simulink model "QpskRxBradeRf"  (R2015b)
settings: Solver=VariableStepAuto  StartTime=0.0  StopTime=inf  RelTol=1e-3
InitFcn:
  | % General simulation parameters
  | M = 4;                         % M-PSK alphabet size
  | Upsampling = 4;            % Upsampling factor
  | Downsampling = 2;        % Downsampling factor
  | Fs = 2e6;                     % Sample rate
  | Ts = 1/Fs;                    % Sample time
  | FrameSize = 111;          % Number of modulated symbols per frame
  | %MessageLength = 105;  % Number of message bits per frame, 7 ASCII characters
  | BarkerLength = 13;        % Number of Barker code symbols
  | 
  | % Rx parameters
  | K = 1;
  | A = 1/sqrt(2);
  | 
  | % TED
  | %fs = 2.4e6;
  | %fs = Fs/2;
  | fs = Fs;
  | Rdata = 100e3;
  | Rsymbol = Rdata/2;
  | 
  | % --- Early Late Timing Synchronisation ----
  | % synch loop design
  | d = 0.707;                   % damping ratio
  | 
  | %Ts = 1/Rsymbol;           % symbol period
  | Ks = 3.22;                    % phase detector coefficient
  | BnS = 0.1*Rsymbol;      % noise bandwidth in Hz
  | Kn   = 1;                      % gain of numerically controlled clock
  | 
  | % calculate loop filter coefficients
  | Ka = (4*d*BnS*Ts)/(Kn*Ks*(d+1/(4*d)));
  | Kb = (4*(BnS*Ts)^2)/(Kn*Ks*(d+1/4*d)^2);
  | 
  | % ------- Carrier Synchronisation --------
  | T = 1/fs;       % sample period
  | Kp = 1;          % phase detector S-curve is linear
  | Bn = 25000;   % noise bandwidth in Hz
  | Ko = 1;          % gain of NCO (here just a direct conversion)
  | 
  | d = 0.707;  % damping ratio
  | 
  | % calculate the loop filter coefficients
  | K1 = (4*d*Bn*T)/(Ko*Kp*(d+1/(4*d)));
  | K2 = (4*(Bn*T)^2)/(Ko*Kp*(d+1/4*d)^2);
libraries: simulink x5, dspstat3 x3, commdigbbndpm3 x2, commrfcorlib x1, commrflib2 x1, commblksprivate x1, dspspect3 x1, commsequence2 x1, dspsigops x1, commutil2 x1, commfilt2 x1
settings Model: ModifiedByFormat=RapidRadio  Creator=RapidRadio  LastModifiedBy=RapidRadio

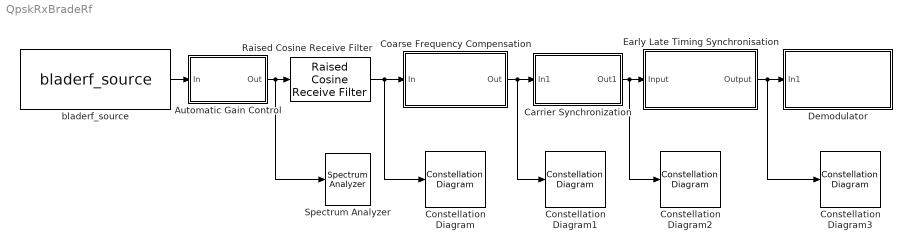
== system QpskRxBradeRf ==
  Automatic Gain Control : Subsystem  mask{DesiredAmplitude=1/sqrt(Upsampling)}
      mask prompts: DesiredAmplitude "Desired Amplitude"
      mask Display: disp('Automatic Gain\nControl')
  Carrier Synchronization : Subsystem
      mask Display: disp('Carrier\nSynchronization');
  Coarse Frequency Compensation : Subsystem
      mask Display: disp('Coarse Frequency\nCompensation');
  Constellation Diagram{,1..3} (4 alike) : ConstellationDiagram
  Demodulator : Subsystem
      mask Display: disp('Demodulator');
  Early Late Timing Synchronisation : Subsystem
      mask Display: disp('Early Late Timing\nSynchronisation');
  Raised Cosine Receive Filter : commfilt2/Raised Cosine Receive Filter  filtType=Square root  N=8  filtSpan=10  currentFiltSpan=10  D=(10)/2  R=0.5  sampMode=Mute  saveAsFlag=0  rateMode=Downsampling  downFactor=8  downOffset=1  framing=Enforce single-rate processing  InputProcessing=Columns as channels (frame based)  checkGain=Normalized  filterGain=1  checkCoeff=off  variableName=rcRxFilt1  launchFVT=off  roundingMode=Floor  overflowMode=off
  Spectrum Analyzer : SpectrumAnalyzer
  bladerf_source : S-Function  FunctionName=bladerf_source  Parameters=set_index,samplerate,set_bandwidth,set_freq,set_lnagain,set_rxvga1,set_rxvga2,set_frame,set_frame_type  SFunctionDeploymentMode=off  EnableBusSupport=off  mask(bladeRF Source){bladerf_device_index=0, bladerf_query=off, bladerf_samplerate=2e6, bladerf_lpf=1.75 MHz, bladerf_frame_length=888, bladerf_frame_type=Frame, bladerf_frequency=2.4e9, bladerf_rxlna=6dB, bladerf_rxvga1=10, bladerf_rxvga2=10, bladerf_restore_block=off}
      mask prompts: bladerf_device_index "Device Index:"; bladerf_query "Find Devices (click, see MATLAB console output)"; bladerf_samplerate "Sample Rate (SPS):"; bladerf_lpf "Low Pass Filter Bandwidth:"; bladerf_frame_length "Samples per frame"; bladerf_frame_type "Output Type:"; bladerf_frequency "Carrier Frequency (Hz):"; bladerf_rxlna "RXLNA Gain (dB)"; bladerf_rxvga1 "RXVGA1 Gain (dB)"; bladerf_rxvga2 "RXVGA2 Gain (dB)"; bladerf_restore_block "Restore Block Size (click)"
      mask help: Receive data from a bladeRF device.
      mask init:
      | % initialize
      | % S-params set_index,samplerate,set_bandwidth,set_freq,set_lnagain,set_rxvga1,set_rxvga2,set_frame,set_frame_type
      | mask_display_text = [];
      | 
      | port=0;
      | % check identifier
      | if (isreal(bladerf_device_index) && bladerf_device_index >= 0)
      |     set_index=bladerf_device_index;
      | else
      |     error('The device index must be a number greater or equal 0 !!!')
      | end
      | 
      | % mask display device index
      | if strcmp(get_param(gcb,'bladerf_device_index'),' ')
      |     mask_display_text = [mask_display_text 'disp(''No Device'');'];
      | else
      |     mask_display_text = [mask_display_text 'disp(''bladeRF #' num2str(bladerf_device_index) ''');'];
      | end
      | if (bladerf_samplerate < bladerf_lpf)
      |     warning('The bandwidth should be lower than the samplerate, use with caution')
      | end
      | % check samplerate
      | if (isreal(bladerf_samplerate))
      |     if (bladerf_samplerate > 0)
      |         samplerate=uint32(bladerf_samplerate);
      |         if (samplerate ~= bladerf_samplerate)
      |             fprintf('Sample Rate adjusted to %u Sps\n',samplerate);
      |         end
      |     else
      |         error('The samplerate has to be greater than 0 !!!')
      |     end
      | else
      |     error('The samplerate has to be number !!!')
      | end
      | 
      | bws = [28e6 20e6 14e6 12e6 8.75e6 7e6 6e6 5.5e6 5e6 3.84e6 3e6 2.75e6 2.5e6 1.75e6 1.5e6];
      | set_bandwidth = bws(bladerf_lpf);
      | if (set_bandwidth > bladerf_samplerate)
      |     warning('Sampling rate (Sps) should be equal to or greater than Low Pass Filter Bandwidth to satisfy Nyquist sampling rate');
      | end
      | 
      | % check frequency
      | if (isreal(bladerf_frequency) && bladerf_frequency >= 0)
      |         set_freq=uint32(bladerf_frequency);
      |         if (set_freq ~= bladerf_frequency)
      |                 fprintf('Frequency adjusted to %d\n',set_freq);
      |         end
      | else
      |     error('The frequency has to be number greater than 0 !!!')
      | end
      | 
      | % LNA gain
      | if (isreal(bladerf_rxlna))
      |     if (bladerf_rxlna == 0)
      |         set_lnagain = 6;
      |     elseif (bladerf_rxlna == 1)
      |         set_lnagain = 3;
      |     else
      |         set_lnagain = 0;
      |     end
      | end
      | 
      | % RXVGA1
      | if (isreal(bladerf_rxvga1))
      |     if (bladerf_rxvga1 < 5)
      |         error('RXVGA1 Gain has to be greater than or equal to 5dB\n');
      |     elseif (bladerf_rxvga1 > 30)
      |         error('RXVGA1 Gain has to be less than or equal to 30dB\n');
      |     else
      |         set_rxvga1 = uint32(bladerf_rxvga1);
      |         if (set_rxvga1 ~= bladerf_rxvga1)
      |             fprintf('RXVGA1 Gain set to %u dB\n', set_rxvga1)
      |         end
      |     end
      | end
      | 
      | % RXVGA2
      | if (isreal(bladerf_rxvga2))
      |     if (bladerf_rxvga2 < 0)
      |         error('RXVGA2 Gain has to be greater than or equal to 0dB\n');
      |     elseif (bladerf_rxvga2 > 30)
      |         error('RXVGA2 Gain has to be less than or equal to 30dB\n');
      |     else
      |         set_rxvga2 = uint32(bladerf_rxvga2);
      |         if (set_rxvga2 ~= bladerf_rxvga2)
      |             fprintf('RXVGA2 Gain set to %u dB\n', set_rxvga2)
      |         end
      |     end
      | end
      | 
      | % check frame length
      | if (isreal(bladerf_frame_length) && bladerf_frame_length > 0)
      |     set_frame=bladerf_frame_length;
      | else
      |     error('The frame length has to be number greater than 0 !!!')
      | end
      | 
      | % check frame type
      | if (strcmp(get_param(gcb,'bladerf_frame_type'),'Frame'))
      |     % use frames
      |     set_frame_type=1;
      | else
      |     % use vectors
      |     set_frame_type=0;
      | end
      |     
      | % set mask display
      | set_param(gcb,'MaskDisplay',mask_display_text);
      mask Help: web(fullfile(bladerf_get_path, 'blockset', 'bladerf_source.html'), '-helpbrowser')
      mask Callback bladerf_query:
      | stat=get_param(gcb,'bladerf_query');
      | set_param(gcb,'bladerf_query','off');
      | 
      | if strcmp(stat,'on')
      |     clear stat;
      |     bladerf_find_devices;
      | end
      | 
      | clear stat;
      mask TypeOptions bladerf_lpf: 28 MHz | 20 MHz | 14 Mhz | 12 Mhz | 8.75 Mhz | 7 MHz | 6 Mhz | 5.5 MHz | 5 MHz | 3.84 MHz | 3 MHz | 2.75 MHz | 2.5 MHz | 1.75 MHz | 1.5 MHz
      mask TypeOptions bladerf_frame_type: Frame | Vector
      mask TypeOptions bladerf_rxlna: 6dB | 3dB | 0dB
      mask Callback bladerf_restore_block:
      | % restore block size
      | block_width=150;
      | block_height=60;
      | 
      | if strcmp(get_param(gcb,'bladerf_restore_block'),'on')
      |    pos=get_param(gcb,'Position');
      |    pos=[pos(1) pos(2) pos(1)+block_width pos(2)+block_height];
      |    set_param(gcb,'Position',pos);
      | end
      | 
      | set_param(gcb,'bladerf_restore_block','off');
      | 
      | clear pos block_width block_height
      mask Display: disp('bladeRF #0');
  wires:
  Raised Cosine Receive Filter/1 -> Constellation Diagram/1, Coarse Frequency Compensation/1(In)
  bladerf_source/1 -> Automatic Gain Control/1(In)
  Coarse Frequency Compensation/1(Out) -> Carrier Synchronization/1(In1), Constellation Diagram1/1
  Early Late Timing Synchronisation/1(Output) -> Demodulator/1(In1), Constellation Diagram3/1
  Automatic Gain Control/1(Out) -> Raised Cosine Receive Filter/1, Spectrum Analyzer/1
  Carrier Synchronization/1(Out1) -> Early Late Timing Synchronisation/1(Input), Constellation Diagram2/1

== system QpskRxBradeRf/Automatic Gain Control ==
  In : Inport
  AGC : commrfcorlib/AGC  LegacyMode=off  DetectorMethod=Rectifier  LoopMethod=Linear  UpdatePeriod=40  StepSize=0.1  AdaptationStepSize=(0.1)/(40)  DesiredOutputPower=1  AveragingLength=40  MaximumGain=1e6  MaxPowerGain=2*(1e6)  GainOutputPort=off  InputPowerOutputPort=off  SimulateUsing=Code generation
  Gain : Gain  Gain=DesiredAmplitude
  Out : Outport
  wires:
  In/1 -> AGC/1
  AGC/1 -> Gain/1
  Gain/1 -> Out/1

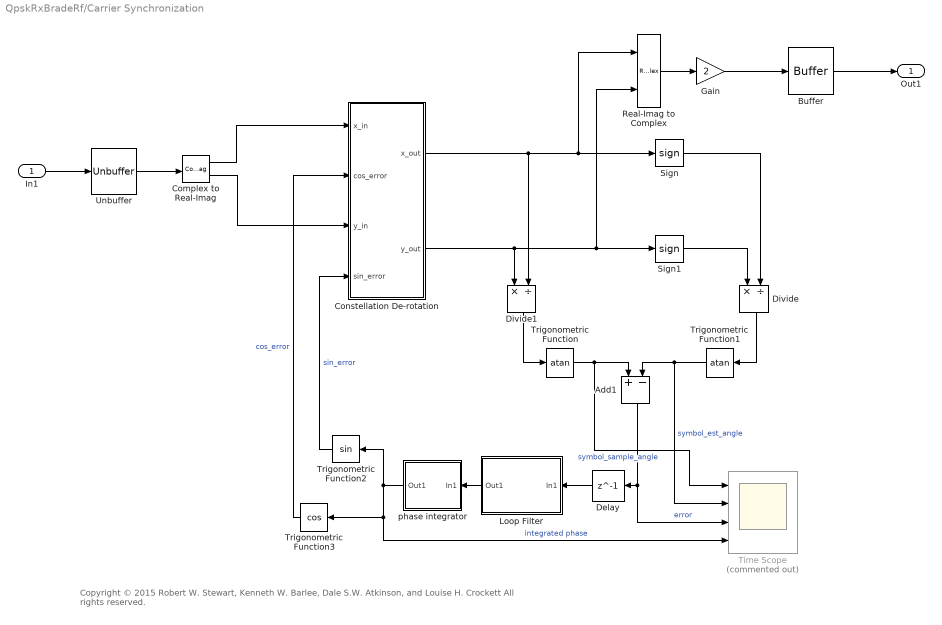
== system QpskRxBradeRf/Carrier Synchronization ==
  note: Copyright © 2015 Robert W. Stewart, Kenneth W. Barlee, Dale S.W. Atkinson, and Louise H. Crockett All rights reserved.
  In1 : Inport
  Add1 : Sum  Inputs=+-
  Buffer : Buffer  N=111  TreatMby1Signals=One channel  OutputFrames=off
  Complex to Real-Imag : ComplexToRealImag
  Constellation De-rotation : Subsystem
  Delay : Delay  DelayLength=1
  Divide : Product  Inputs=*/
  Divide1 : Product  Inputs=*/
  Gain : Gain  Gain=2
  Loop Filter : Subsystem
  Real-Imag to Complex : RealImagToComplex
  Sign : Signum
  Sign1 : Signum
  Time Scope : Scope  Commented=on  NumInputPorts=4
      settings: StartFcn=startfcn_time_scope;
  Trigonometric Function : Trigonometry  Operator=atan  OutputSignalType=real
  Trigonometric Function1 : Trigonometry  Operator=atan  OutputSignalType=real
  Trigonometric Function2 : Trigonometry
  Trigonometric Function3 : Trigonometry  Operator=cos
  Unbuffer : Unbuffer  SampleBasedProcessing=Same as frame based
  phase integrator : Subsystem
  Out1 : Outport
  wires:
  Real-Imag to Complex/1 -> Gain/1
  Sign1/1 -> Divide/1
  Sign/1 -> Divide/2
  Constellation De-rotation/2(y_out) -> Sign1/1, Real-Imag to Complex/2, Divide1/1
  Divide/1 -> Trigonometric Function1/1
  Delay/1 -> Loop Filter/1(In1)
  Divide1/1 -> Trigonometric Function/1
  Add1/1 -> Time Scope/3, Delay/1  "error"
  Constellation De-rotation/1(x_out) -> Sign/1, Real-Imag to Complex/1, Divide1/2
  phase integrator/1(Out1) -> Trigonometric Function2/1, Time Scope/4, Trigonometric Function3/1  "integrated phase"
  Trigonometric Function1/1 -> Time Scope/2, Add1/2  "symbol_est_angle"
  Trigonometric Function/1 -> Add1/1, Time Scope/1  "symbol_sample_angle"
  Trigonometric Function2/1 -> Constellation De-rotation/4(sin_error)  "sin_error"
  Trigonometric Function3/1 -> Constellation De-rotation/2(cos_error)  "cos_error"
  Loop Filter/1(Out1) -> phase integrator/1(In1)
  Complex to Real-Imag/1 -> Constellation De-rotation/1(x_in)
  Complex to Real-Imag/2 -> Constellation De-rotation/3(y_in)
  In1/1 -> Unbuffer/1
  Unbuffer/1 -> Complex to Real-Imag/1
  Gain/1 -> Buffer/1
  Buffer/1 -> Out1/1

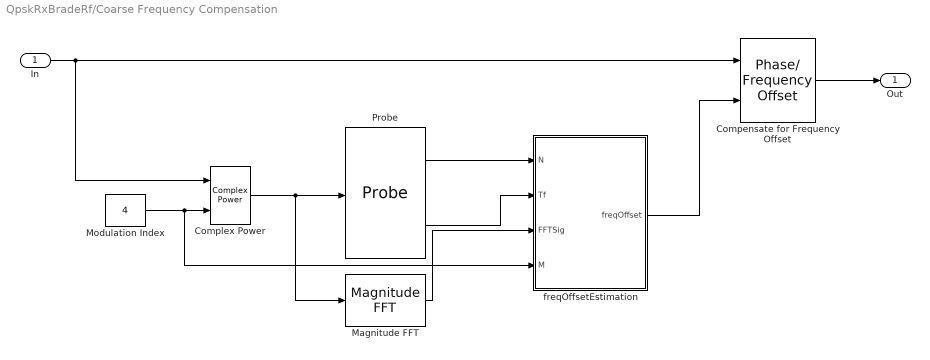
== system QpskRxBradeRf/Coarse Frequency Compensation ==
  In : Inport
  Compensate for Frequency Offset : commrflib2/Phase// Frequency Offset  phaseOffset=0  freqPort=on  freqOffset=100
  Complex Power : commblksprivate/Complex Power
  Magnitude FFT : dspspect3/Magnitude FFT  mag_or_magsq=Magnitude squared  FFTImplementation=Auto  fftLenInherit=on  fftsize=1024  WrapInput=on
  Modulation Index : Constant  Value=4  OutDataTypeStr=Inherit: Inherit via back propagation
  Probe : Probe  ProbeComplexSignal=off
  freqOffsetEstimation : MATLAB Function  TreatAsAtomicUnit=on
  Out : Outport
  wires:
  Compensate for Frequency Offset/1 -> Out/1
  freqOffsetEstimation/1(freqOffset) -> Compensate for Frequency Offset/2
  Magnitude FFT/1 -> freqOffsetEstimation/3(FFTSig)
  Modulation Index/1 -> freqOffsetEstimation/4(M), Complex Power/2
  Probe/1 -> freqOffsetEstimation/1(N)
  Probe/2 -> freqOffsetEstimation/2(Tf)
  Complex Power/1 -> Magnitude FFT/1, Probe/1
  In/1 -> Complex Power/1, Compensate for Frequency Offset/1

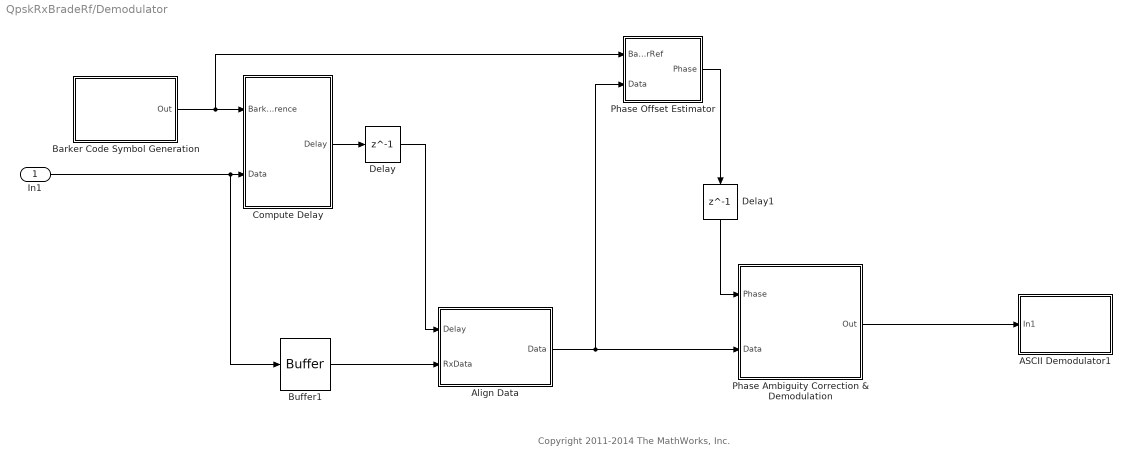
== system QpskRxBradeRf/Demodulator ==
  note: Copyright 2011-2014 The MathWorks, Inc.
  In1 : Inport
  ASCII Demodulator1 : Subsystem
      mask Display: disp('ASCII Demodulator')
  Align Data : MATLAB Function  TreatAsAtomicUnit=on
  "Barker Code Symbol Generation " : Subsystem
      mask Display: disp('Barker Code\nSymbol Generation')
  Buffer1 : Buffer  N=FrameSize*2  V=FrameSize  TreatMby1Signals=One channel
  Compute Delay : Subsystem
      mask Display: disp('Compute\nDelay');
  Delay : Delay  DelayLength=1
  Delay1 : Delay  DelayLength=1
  Phase Ambiguity Correction & Demodulation : Subsystem
      mask Display: disp('Phase Ambiguity\nCorrection\n& Demodulation');
  Phase Offset Estimator : Subsystem
  wires:
  In1/1 -> Buffer1/1, Compute Delay/2(Data)
  Delay/1 -> Align Data/1(Delay)
  Compute Delay/1(Delay) -> Delay/1
  Align Data/1(Data) -> Phase Ambiguity Correction & Demodulation/2(Data), Phase Offset Estimator/2(Data)
  "Barker Code Symbol Generation "/1(Out) -> Compute Delay/1(Barker Reference), Phase Offset Estimator/1(BarkerRef)
  Buffer1/1 -> Align Data/2(RxData)
  Phase Offset Estimator/1(Phase) -> Delay1/1
  Delay1/1 -> Phase Ambiguity Correction & Demodulation/1(Phase)
  Phase Ambiguity Correction & Demodulation/1(Out) -> ASCII Demodulator1/1(In1)

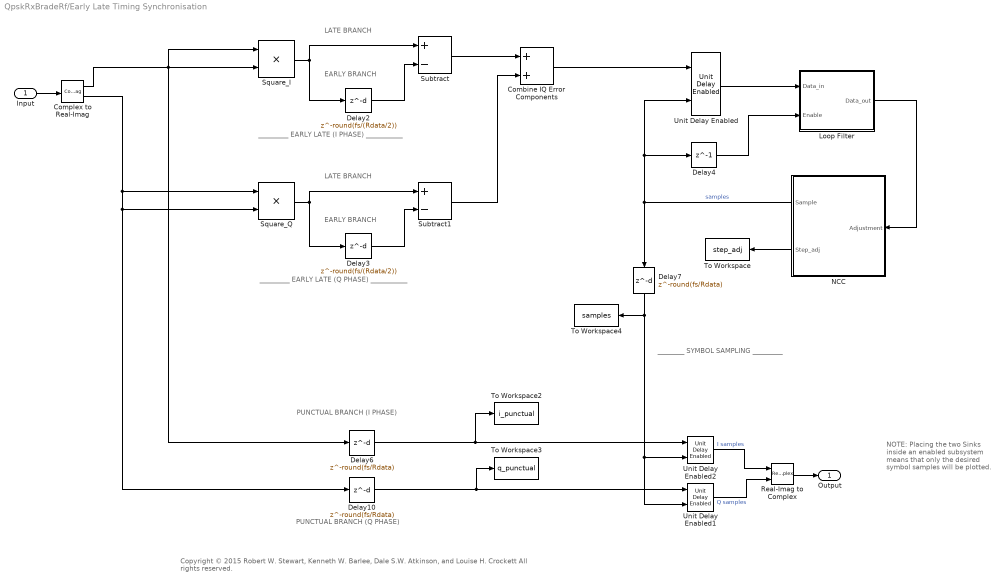
== system QpskRxBradeRf/Early Late Timing Synchronisation ==
  note: NOTE:
      |
      | Placing the two Sinks inside an
      | enabled subsystem means that
      | only the desired symbol samples
      | will be plotted.
  note: LATE BRANCH
  note: EARLY BRANCH
  note: PUNCTUAL BRANCH (I PHASE)
  note: LATE BRANCH
  note: EARLY BRANCH
  note: _________ EARLY LATE (I PHASE) ___________
  note: _________ EARLY LATE (Q PHASE) ___________
  note: ________ SYMBOL SAMPLING _________
  note: PUNCTUAL BRANCH (Q PHASE)
  note: Copyright © 2015 Robert W. Stewart, Kenneth W. Barlee, Dale S.W. Atkinson, and Louise H. Crockett All rights reserved.
  Input : Inport
  Combine IQ Error Components : Sum
  Complex to Real-Imag : ComplexToRealImag
  Delay10 : Delay  DelayLength=round(fs/Rdata)
  Delay2 : Delay  DelayLength=round(fs/(Rdata/2))
  Delay3 : Delay  DelayLength=round(fs/(Rdata/2))
  Delay4 : Delay  DelayLength=1
  Delay6 : Delay  DelayLength=round(fs/Rdata)
  Delay7 : Delay  DelayLength=round(fs/Rdata)
  Loop Filter : Subsystem
  NCC : Subsystem  mask(Numerically Controller Clock (NCC)){OSR=fs/Rsymbol}
      mask prompts: OSR "Oversampling Ratio"
      mask help:
      | This component operates similarly to a Numerically Controlled Oscillator (NCO).
      |
      | Internally, a nominal step size of (1 + Adjustment) is applied to an accumulator. The accumulator wraps around at N = OSR, therefore for a zero control input, the accumulator wraps once every symbol period at the expected rate.
      |
      | When the accumulator wraps, a strobe output is produced.
  Real-Imag to Complex : RealImagToComplex
  Square_I : Product
  Square_Q : Product
  Subtract : Sum  Inputs=+-
  Subtract1 : Sum  Inputs=+-
  To Workspace : ToWorkspace  VariableName=step_adj  SaveFormat=Structure With Time  SampleTime=-1
  To Workspace2 : ToWorkspace  VariableName=i_punctual  SaveFormat=Structure With Time  SampleTime=-1
  To Workspace3 : ToWorkspace  VariableName=q_punctual  SaveFormat=Structure With Time  SampleTime=-1
  To Workspace4 : ToWorkspace  VariableName=samples  SaveFormat=Structure With Time  SampleTime=-1
  Unit Delay Enabled : simulink/Additional Math & Discrete/Additional Discrete/Unit Delay Enabled  vinit=0.0  tsamp=-1
  Unit Delay Enabled1 : simulink/Additional Math & Discrete/Additional Discrete/Unit Delay Enabled  vinit=0.0  tsamp=-1
  Unit Delay Enabled2 : simulink/Additional Math & Discrete/Additional Discrete/Unit Delay Enabled  vinit=0.0  tsamp=-1
  Output : Outport
  wires:
  Subtract/1 -> Combine IQ Error Components/1
  Delay4/1 -> Loop Filter/2(Enable)
  Square_Q/1 -> Delay3/1, Subtract1/1
  Square_I/1 -> Subtract/1, Delay2/1
  Delay2/1 -> Subtract/2
  Unit Delay Enabled/1 -> Loop Filter/1(Data_in)
  NCC/1(Sample) -> Unit Delay Enabled/2, Delay4/1, Delay7/1  "samples"
  Loop Filter/1(Data_out) -> NCC/1(Adjustment)
  Subtract1/1 -> Combine IQ Error Components/2
  Complex to Real-Imag/1 -> Square_I/1, Delay6/1, Square_I/2
  Delay6/1 -> To Workspace2/1, Unit Delay Enabled2/1
  Delay3/1 -> Subtract1/2
  Unit Delay Enabled2/1 -> Real-Imag to Complex/1  "I samples"
  NCC/2(Step_adj) -> To Workspace/1
  Combine IQ Error Components/1 -> Unit Delay Enabled/1
  Unit Delay Enabled1/1 -> Real-Imag to Complex/2  "Q samples"
  Delay10/1 -> To Workspace3/1, Unit Delay Enabled1/1
  Complex to Real-Imag/2 -> Delay10/1, Square_Q/2, Square_Q/1
  Delay7/1 -> Unit Delay Enabled2/2, Unit Delay Enabled1/2, To Workspace4/1
  Input/1 -> Complex to Real-Imag/1
  Real-Imag to Complex/1 -> Output/1

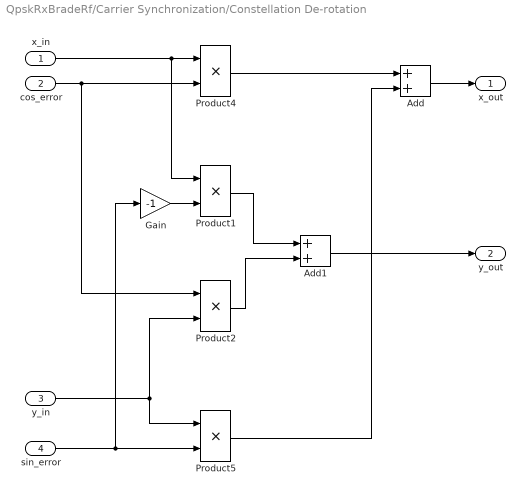
== system QpskRxBradeRf/Carrier Synchronization/Constellation De-rotation ==
  x_in : Inport
  cos_error : Inport  Port=2
  y_in : Inport  Port=3
  sin_error : Inport  Port=4
  Add : Sum
  Add1 : Sum
  Gain : Gain  Gain=-1
  Product{1..2,4..5} (4 alike) : Product
  x_out : Outport
  y_out : Outport  Port=2
  wires:
  Product4/1 -> Add/1
  y_in/1 -> Product2/2, Product5/1
  sin_error/1 -> Gain/1, Product5/2
  x_in/1 -> Product1/1, Product4/1
  Product5/1 -> Add/2
  cos_error/1 -> Product2/1, Product4/2
  Add/1 -> x_out/1
  Gain/1 -> Product1/2
  Product2/1 -> Add1/2
  Product1/1 -> Add1/1
  Add1/1 -> y_out/1

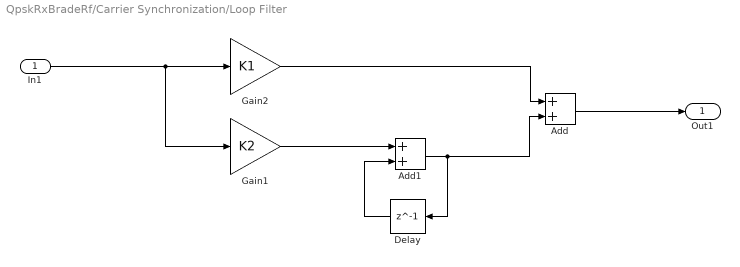
== system QpskRxBradeRf/Carrier Synchronization/Loop Filter ==
  In1 : Inport
  Add : Sum
  Add1 : Sum
  Delay : Delay  DelayLength=1
  Gain1 : Gain  Gain=K2
  Gain2 : Gain  Gain=K1
  Out1 : Outport
  wires:
  Add/1 -> Out1/1
  Gain2/1 -> Add/1
  Delay/1 -> Add1/2
  Add1/1 -> Delay/1, Add/2
  Gain1/1 -> Add1/1
  In1/1 -> Gain1/1, Gain2/1

== system QpskRxBradeRf/Carrier Synchronization/phase integrator ==
  In1 : Inport
  Add1 : Sum
  Delay : Delay  DelayLength=1
  Gain2 : Gain  Gain=Ko
  Out1 : Outport
  wires:
  In1/1 -> Add1/1
  Add1/1 -> Gain2/1, Delay/1
  Delay/1 -> Add1/2
  Gain2/1 -> Out1/1

== system QpskRxBradeRf/Demodulator/ASCII Demodulator1 ==
  In1 : Inport
  Descrambler : commsequence2/Descrambler  M=2  poly=[1 1 1 0 1]  iniStaSource=Dialog Parameter  ini_sta=[0 0 0 0]  resetViaPort=off
  MATLAB Function : MATLAB Function  TreatAsAtomicUnit=on
  Selector : Selector  InputPortWidth=222  IndexOptions=Index vector (dialog)  Indices=[27:208]  OutputSizes=1
  wires:
  In1/1 -> Selector/1
  Descrambler/1 -> MATLAB Function/1(u)
  Selector/1 -> Descrambler/1

== system QpskRxBradeRf/Demodulator/Barker Code Symbol Generation  ==
  note: Regenerate a QPSK-modulated unipolar Barker code sequence
      | to be compared with the received data
  Constant Barker Code : Constant  Value=|  VectorParams1D=off
      | [+1 +1 +1 +1 +1 -1 -1 +1 +1 -1 +1 -1 +1
      | ].' > 0
      settings: SamplingMode=Frame based
  Data Type Conversion : DataTypeConversion  OutDataTypeStr=double
  QPSK Modulator Baseband : commdigbbndpm3/QPSK Modulator Baseband  InType=Bit  Enc=Gray  Ph=pi/4  outDtype=double  outWordLen=16  outUDDataType=sfix(16)  outFracLenMode=Best precision  outFracLen=15
  Repeat : dspsigops/Repeat  N=2  InputProcessing=Columns as channels (frame based)  RateOptions=Enforce single-rate processing  ic=0  mode=Unused parameter value
  Out : Outport
  wires:
  Constant Barker Code/1 -> Data Type Conversion/1
  Repeat/1 -> QPSK Modulator Baseband/1
  QPSK Modulator Baseband/1 -> Out/1
  Data Type Conversion/1 -> Repeat/1

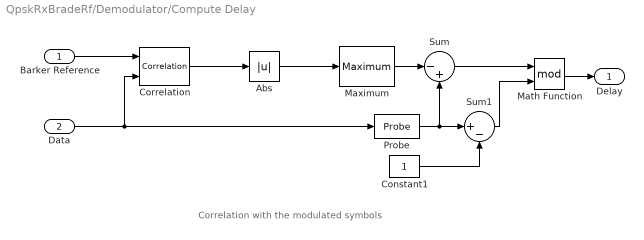
== system QpskRxBradeRf/Demodulator/Compute Delay ==
  note: Correlation with the modulated symbols
  Barker Reference : Inport
  Data : Inport  Port=2
  Abs : Abs
  Constant1 : Constant  VectorParams1D=off  OutDataTypeStr=Inherit: Inherit via back propagation  FramePeriod=2
  Correlation : dspstat3/Correlation  domain=Time  outputDataTypeStr=Inherit: Same as accumulator  outputLastDataTypeStr=Inherit: Same as accumulator  outputMin=[]  outputMax=[]  accumDataTypeStr=Inherit: Same as product output  accumLastDataTypeStr=Inherit: Same as product output  roundingMode=Floor  overflowMode=off
  Math Function : Math  Operator=mod  SaturateOnIntegerOverflow=on
  Maximum : dspstat3/Maximum  fcn=Index  reset=None  InputProcessing=Columns as channels (frame based)  indexBase=One  operateOver=Each column  Dimension=1  operation=maximum  roiEnable=off  roiType=Rectangles  roiPortion=Entire ROI  roiOutput=Individual statistics for each ROI  roiFlag=off  accumDataTypeStr=Inherit: Same as product output  accumLastDataTypeStr=Inherit: Same as product output  roundingMode=Floor  overflowMode=off
  Probe : Probe  ProbeSampleTime=off  ProbeComplexSignal=off
  Sum : Sum  Inputs=|-+  SaturateOnIntegerOverflow=on  InputSameDT=on  OutDataTypeStr=Inherit: Same as first input
  Sum1 : Sum  Inputs=|+-  SaturateOnIntegerOverflow=on  InputSameDT=on  OutDataTypeStr=Inherit: Same as first input
  Delay : Outport
  wires:
  Abs/1 -> Maximum/1
  Constant1/1 -> Sum1/2
  Sum1/1 -> Math Function/2
  Math Function/1 -> Delay/1
  Sum/1 -> Math Function/1
  Probe/1 -> Sum1/1, Sum/2
  Correlation/1 -> Abs/1
  Maximum/1 -> Sum/1
  Barker Reference/1 -> Correlation/1
  Data/1 -> Correlation/2, Probe/1

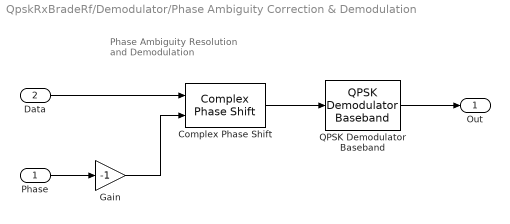
== system QpskRxBradeRf/Demodulator/Phase Ambiguity Correction & Demodulation ==
  note: Phase Ambiguity Resolution
      | and Demodulation
  Phase : Inport
  Data : Inport  Port=2
  Complex Phase Shift : commutil2/Complex Phase Shift
  Gain : Gain  Gain=-1
  QPSK Demodulator Baseband : commdigbbndpm3/QPSK Demodulator Baseband  Ph=pi/4  Dec=Gray  OutType=Bit  DecType=Hard decision  VarSource=Dialog  Variance=1  outDtype1=Inherit via internal rule  outDtype2=Inherit via internal rule  derotateFactorWordLen=16
  Out : Outport
  wires:
  Phase/1 -> Gain/1
  Data/1 -> Complex Phase Shift/1
  Complex Phase Shift/1 -> QPSK Demodulator Baseband/1
  QPSK Demodulator Baseband/1 -> Out/1
  Gain/1 -> Complex Phase Shift/2

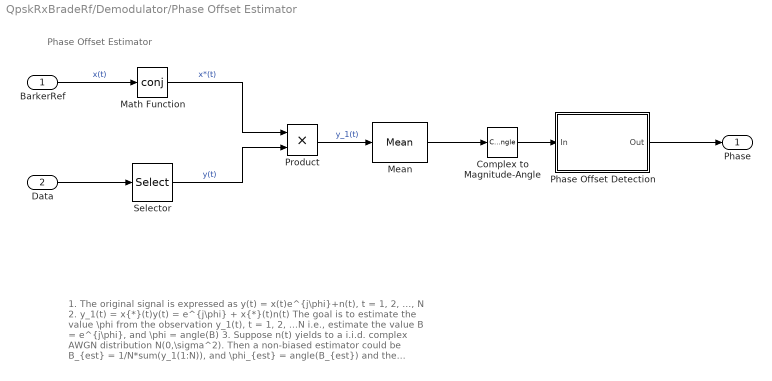
== system QpskRxBradeRf/Demodulator/Phase Offset Estimator ==
  note: Phase Offset Estimator
  note: 1. The original signal is expressed as y(t) = x(t)e^{j\phi}+n(t), t = 1, 2, ..., N
      | 2. y_1(t) = x{*}(t)y(t) = e^{j\phi} + x{*}(t)n(t)
      | The goal is to estimate the value \phi from the observation y_1(t), t = 1, 2, ...N
      | i.e., estimate the value B = e^{j\phi}, and \phi = angle(B)
      | 3. Suppose n(t) yields to a i.i.d. complex AWGN distribution N(0,\sigma^2).
      | Then a non-biased estimator could be
      | B_{est} = 1/N*sum(y_1(1:N)), and \phi_{est} = angle(B_{est})
      | and the variance of B_{est} is \sigma^2/N
  BarkerRef : Inport
  Data : Inport  Port=2
  Complex to Magnitude-Angle : ComplexToMagnitudeAngle  Output=Angle
  Math Function : Math  Operator=conj  SaturateOnIntegerOverflow=on
  Mean : dspstat3/Mean  run=off  reset_popup=None  InputProcessing=Columns as channels (frame based)  directionMode=Each column  dimension=1  roiEnable=off  roiType=Rectangles  roiPortion=Entire ROI  roiOutput=Individual statistics for each ROI  roiFlag=off  outputDataTypeStr=Inherit: Same as accumulator  outputLastDataTypeStr=Inherit: Same as accumulator  outputMin=[]  outputMax=[]  roundingMode=Floor  overflowMode=off
  Phase Offset Detection : MATLAB Function  TreatAsAtomicUnit=on
  Product : Product  RndMeth=Zero
  Selector : Selector  IndexOptions=Index vector (dialog)  Indices=[1:BarkerLength]  OutputSizes=1
  Phase : Outport
  wires:
  Data/1 -> Selector/1
  BarkerRef/1 -> Math Function/1  "x(t)"
  Selector/1 -> Product/2  "y(t)"
  Math Function/1 -> Product/1  "x*(t)"
  Product/1 -> Mean/1  "y_1(t)"
  Mean/1 -> Complex to Magnitude-Angle/1
  Complex to Magnitude-Angle/1 -> Phase Offset Detection/1(In)
  Phase Offset Detection/1(Out) -> Phase/1

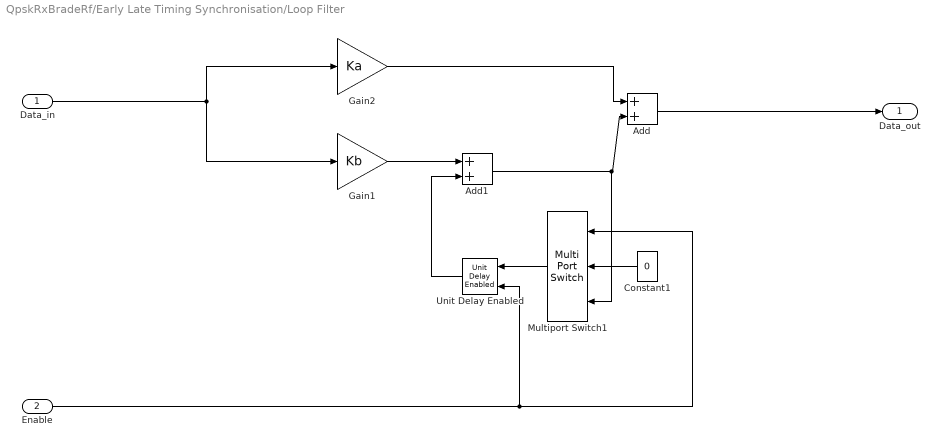
== system QpskRxBradeRf/Early Late Timing Synchronisation/Loop Filter ==
  Data_in : Inport
  Enable : Inport  Port=2
  Add : Sum
  Add1 : Sum
  Constant1 : Constant  Value=0  SampleTime=1/fs
  Gain1 : Gain  Gain=Kb
  Gain2 : Gain  Gain=Ka
  Multiport Switch1 : MultiPortSwitch  DataPortOrder=Zero-based contiguous  Inputs=2
  Unit Delay Enabled : simulink/Additional Math & Discrete/Additional Discrete/Unit Delay Enabled  vinit=0.0  tsamp=-1
  Data_out : Outport
  wires:
  Gain1/1 -> Add1/1
  Gain2/1 -> Add/1
  Unit Delay Enabled/1 -> Add1/2
  Add1/1 -> Multiport Switch1/3, Add/2
  Data_in/1 -> Gain2/1, Gain1/1
  Add/1 -> Data_out/1
  Enable/1 -> Unit Delay Enabled/2, Multiport Switch1/1
  Multiport Switch1/1 -> Unit Delay Enabled/1
  Constant1/1 -> Multiport Switch1/2

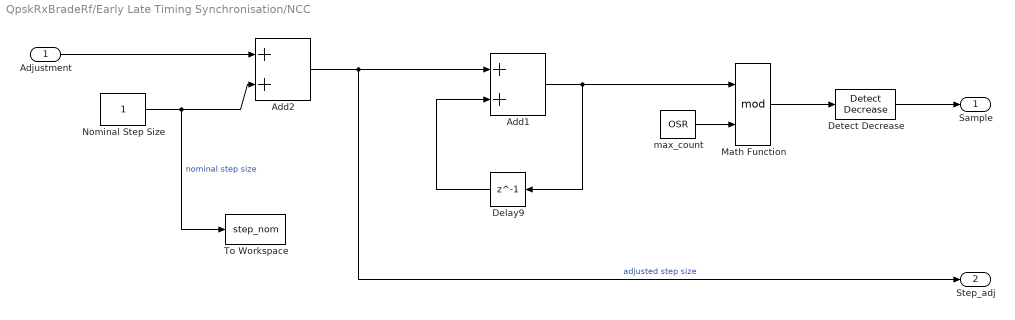
== system QpskRxBradeRf/Early Late Timing Synchronisation/NCC ==
  Adjustment : Inport
  Add1 : Sum  OutDataTypeStr=double
  Add2 : Sum  OutDataTypeStr=double
  Delay9 : Delay  DelayLength=1
  Detect Decrease : simulink/Logic and Bit Operations/Detect Decrease  vinit=0.0  InputProcessing=Inherited  OutDataTypeStr=boolean
  Math Function : Math  Operator=mod  SaturateOnIntegerOverflow=on
  Nominal Step Size : Constant  OutDataTypeStr=double  SampleTime=1/fs
  To Workspace : ToWorkspace  VariableName=step_nom  SaveFormat=Structure With Time  SampleTime=-1
  max_count : Constant  Value=OSR  OutDataTypeStr=double  SampleTime=1/fs
  Sample : Outport
  Step_adj : Outport  Port=2
  wires:
  Adjustment/1 -> Add2/1
  Add2/1 -> Step_adj/1, Add1/1  "adjusted step size"
  Delay9/1 -> Add1/2
  Nominal Step Size/1 -> To Workspace/1, Add2/2  "nominal step size"
  Add1/1 -> Delay9/1, Math Function/1
  Math Function/1 -> Detect Decrease/1
  max_count/1 -> Math Function/2
  Detect Decrease/1 -> Sample/1

== matlab function QpskRxBradeRf/Coarse Frequency Compensation/freqOffsetEstimation ==
  data: N input; freqOffset output; Tf input; FFTSig input; M input
%% Frequency offset estimation
function freqOffset = fcn(N,Tf,FFTSig,M)
[~,maxIdx] = max(FFTSig);
FFTSize = size(FFTSig,1);
if maxIdx > FFTSize/2
    OffsetIdx = FFTSize+1-maxIdx;
else
    OffsetIdx = 1-maxIdx;
end
% Map offset index to a frequency value.
% Compute offset using modulation alphabet size params.M.
Ts = Tf(1)/N; % Sample time
delta_f = 1/(Ts*FFTSize); % Frequency resolution of FFT
freqOffset = OffsetIdx * delta_f / M;

== matlab function QpskRxBradeRf/Demodulator/Align Data ==
  data: Delay input; RxData input; Data output
function Data  = aligndata(Delay, RxData)
% Extract data from the buffered RxData, using the delay to find the frame 
% start
%
% Input:
% Delay - Index of frame start
% RxData - Buffered symbol-spaced data
% Output:
% Data - Data with the Barker code at frame start
%#codegen
Data = RxData(Delay+1:Delay+length(RxData)/2);

== matlab function QpskRxBradeRf/Demodulator/ASCII Demodulator1/MATLAB Function ==
  data: u input
function bitDemod(u)
%#codegen

weight = [int8(64) int8(32) int8(16) int8(8) int8(4) int8(2) int8(1)];
reshaped = reshape(u, [], 7);
weight = repmat(weight, [numel(reshaped)/7 1]);
decimal = weight.*int8(reshaped);
decimal = sum(decimal, 2);
disp(char(decimal'));

== matlab function QpskRxBradeRf/Demodulator/Phase Offset Estimator/Phase Offset Detection ==
  data: In input; Out output
function Out = phasedecision(In)
% Map the estimated phase to one of -pi, -pi/2, 0, pi/2,  
%#codegen
% Out = round(In.*2./pi)./2.*pi;
% The above processing is equivalent to the following processing using
% if/else statements
%
% if In<pi/4 && In>-pi/4
%     Out = 0;
% elseif In>=pi/4 && In<pi*3/4
%     Out = pi/2;
% elseif In>=pi*3/4 || In<=-pi*3/4
%     Out = -pi;
% else
%     Out = -pi/2;
% end

if In<pi/4 && In>=-pi/4
    Out = 0;
elseif In>=pi/4 && In<pi*3/4
    Out = pi/2;
elseif In>=pi*3/4 || In<-pi*3/4
    Out = -pi;
else
    Out = -pi/2;
end
